simulink model "implementation_deploy_mpc"  (R2024a)
settings: configuration reference "Configuration" (kept outside this file)
undefined symbols (not defined in the file): aceleracao_lateral_max, constans_PID, desired_x, desired_y, max_velocity_longitudinal, pos_theta, pos_x, pos_y, PredictionHorizon, Ts, vel_x
libraries: canmsglib x3, nvidiaCommlib x3, ros2lib x2, svdutilitieslib x1, mpcadaslib x1, drivingvehiclecontroller x1, slpidlib x1
settings Model: DataDictionary=implementacao_deploy.sldd  Creator=helenamandl  LastModifiedBy=thailon
settings ConfigSetRef: SourceName=Configuration

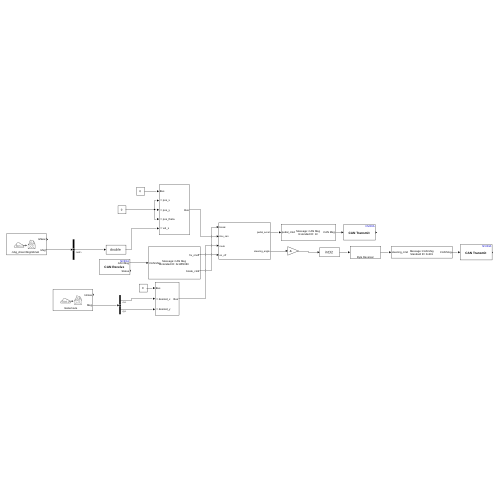
[thumbnail: Simulink's stored preview of the top-level diagram]
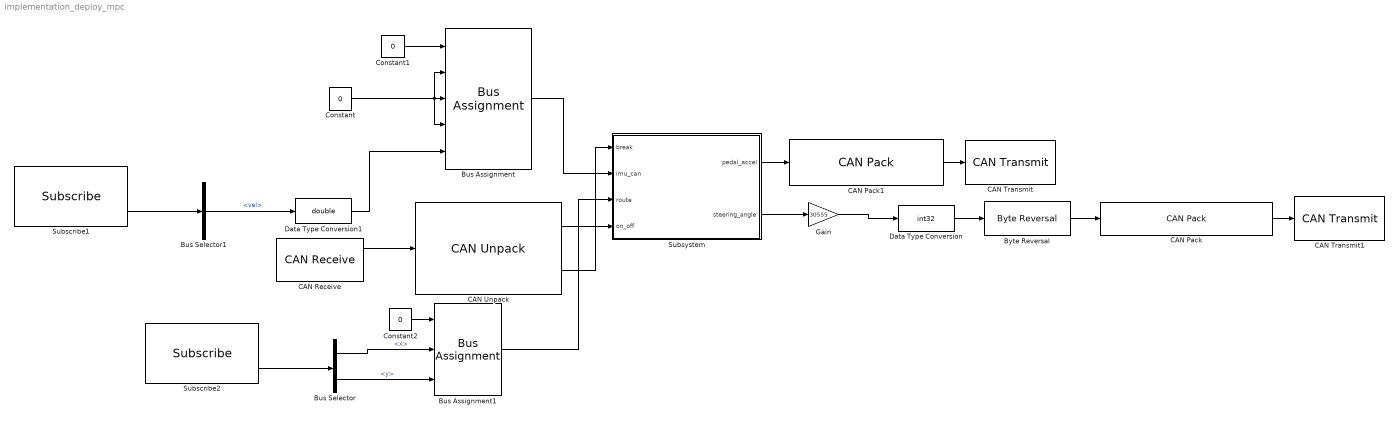
== system implementation_deploy_mpc ==
  Bus Assignment : BusAssignment  AssignedSignals=pos_x,pos_y,pos_theta,vel_x
  Bus Assignment1 : BusAssignment  AssignedSignals=desired_x,desired_y
  Bus Selector : BusSelector  OutputSignals=pose.position.x,pose.position.y
  Bus Selector1 : BusSelector  OutputSignals=vel
  Byte Reversal : svdutilitieslib/Byte Reversal  numInp=1  blockPlatform=arduinoert
      settings: LibrarySourceBlock=mcblib/Signal Management/Byte Reversal
  CAN Pack : canmsglib/CAN Pack  MsgList=(none)  MsgName=CAN Msg  MsgIDType=Standard (11-bit identifier)  MsgIdentifier=0x401  MsgLength=4  Remote=off  ApplyMinMax=off  BusOutput=on  SignalInfo={ 'steering_cmd', '0', '32', 'LE', 'signed', 'Standard', '0', '1', '0', '-Inf', 'Inf' }
      settings: LibrarySourceBlock=c2000lib/Target Communication/CAN Pack  DataFormat=manually specified signals
  CAN Pack1 : canmsglib/CAN Pack  MsgList=(none)  MsgName=CAN Msg  MsgIDType=Extended (29-bit identifier)  MsgIdentifier=13  MsgLength=1  Remote=off  ApplyMinMax=off  BusOutput=on  SignalInfo={ 'pedal_cmd', '0', '8', 'LE', 'unsigned', 'Standard', '0', '1', '0', '0', '100' }
      settings: LibrarySourceBlock=c2000lib/Target Communication/CAN Pack  DataFormat=manually specified signals
  CAN Receive : nvidiaCommlib/CAN Receive  DeviceID=can0  SetupCAN=off  TypeofCAN=Real  OutputDataType=CAN Msg  IdentifierType=Extended (29-bit identifier)  MessageId=0x18ff1080  MsgLength=8  SampleTime=0.005  OutputError=off  OutputRemote=off  SimulateUsing=Code generation
  CAN Transmit : nvidiaCommlib/CAN Transmit  DeviceID=vcan0  SetupCAN=off  TypeofCAN=Real  InputDataType=CAN Msg  BlockingMode_=off  BlockTimeout_=1  OutputStatus=on  IdentifierType=Standard (11-bit identifier)  MessageId=13  MsgLength=8  RemoteFrame=off  SimulateUsing=Code generation
  CAN Transmit1 : nvidiaCommlib/CAN Transmit  DeviceID=vcan0  SetupCAN=off  TypeofCAN=Real  InputDataType=CAN Msg  BlockingMode_=off  BlockTimeout_=1  OutputStatus=on  IdentifierType=Extended (29-bit identifier)  MessageId=0x401  MsgLength=4  RemoteFrame=off  SimulateUsing=Code generation
  CAN Unpack : canmsglib/CAN Unpack  MsgList=(none)  MsgName=CAN Msg  MsgIDType=Extended (29-bit identifier)  MsgIdentifier=0x18ff1080  MsgLength=4  SignalInfo={ 'hv_onoff', '0', '2', 'LE', 'signed', 'Standard', '0', '1', '0', '0', '3'; 'break_cmd', '3', '8', 'LE', 'signed', 'Standard', '1', '1', '0', '0', '255' }  IDPort=off  TimestampPort=off  ErrorPort=off  RemotePort=off  LengthPort=off  StatusPort=off  ApplyMinMax=off
      settings: LibrarySourceBlock=embeddedtargetslib/Host Communication/CAN Unpack
  Constant : Constant  Value=0
  Constant1 : Constant  Value=0  OutDataTypeStr=Bus: bus_imu
  Constant2 : Constant  Value=0  OutDataTypeStr=Bus: bus_route
  Data Type Conversion : DataTypeConversion  OutDataTypeStr=int32  SaturateOnIntegerOverflow=off  RndMeth=Floor
  Data Type Conversion1 : DataTypeConversion  OutDataTypeStr=double  SaturateOnIntegerOverflow=off  RndMeth=Floor
  Gain : Gain  Gain=30555
  Subscribe1 : ros2lib/Subscribe  topicSource=Specify your own  topic=/sbg_driver/SbgOdoVel  messageType=sbg_driver/SbgOdoVel  sampleTime=ts_ros2  QOSHistory=Keep last  QOSDepth=10  QOSReliability=Reliable  QOSDurability=Volatile  QOSDeadline=Inf  QOSLifespan=Inf  QOSLiveliness=Automatic  QOSLeaseDuration=Inf  QOSAvoidROSNamespaceConventions=off
  Subscribe2 : ros2lib/Subscribe  topicSource=Specify your own  topic=/teste/route  messageType=geometry_msgs/PoseStamped  sampleTime=ts_ros2  QOSHistory=Keep last  QOSDepth=10  QOSReliability=Reliable  QOSDurability=Volatile  QOSDeadline=Inf  QOSLifespan=Inf  QOSLiveliness=Automatic  QOSLeaseDuration=Inf  QOSAvoidROSNamespaceConventions=off
  Subsystem : Subsystem
  wires:
  CAN Pack/1 -> CAN Transmit1/1
  Data Type Conversion/1 -> Byte Reversal/1
  Subsystem/1(pedal_accel) -> CAN Pack1/1
  Bus Assignment1/1 -> Subsystem/3(route)
  CAN Unpack/1 -> Subsystem/4(on_off)
  Bus Assignment/1 -> Subsystem/2(imu_can)
  Byte Reversal/1 -> CAN Pack/1
  Bus Selector/2 -> Bus Assignment1/3  "<y>"
  Subscribe1/2 -> Bus Selector1/1
  Bus Selector1/1 -> Data Type Conversion1/1  "<vel>"
  CAN Pack1/1 -> CAN Transmit/1
  Constant2/1 -> Bus Assignment1/1
  CAN Unpack/2 -> Subsystem/1(break)
  Subscribe2/2 -> Bus Selector/1
  Gain/1 -> Data Type Conversion/1
  Subsystem/2(steering_angle) -> Gain/1
  Data Type Conversion1/1 -> Bus Assignment/5
  Bus Selector/1 -> Bus Assignment1/2  "<x>"
  Constant1/1 -> Bus Assignment/1
  CAN Receive/1 -> CAN Unpack/1
  Constant/1 -> Bus Assignment/2, Bus Assignment/4, Bus Assignment/3

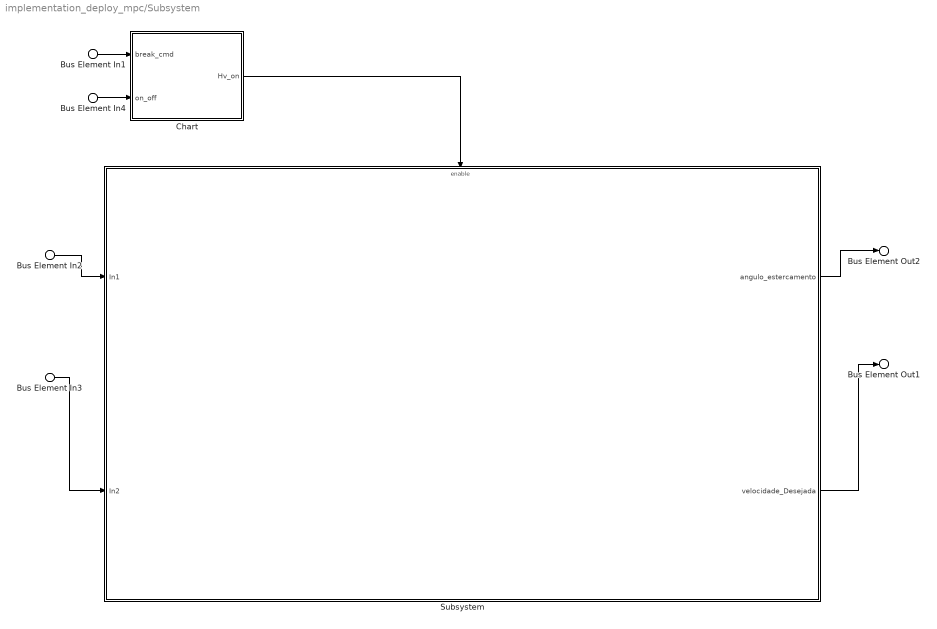
== system implementation_deploy_mpc/Subsystem ==
  Bus Element In1 : Inport  PortName=break
  Bus Element In2 : Inport  Port=2  PortName=imu_can
  Bus Element In3 : Inport  Port=3  PortName=route
  Bus Element In4 : Inport  Port=4  PortName=on_off
  Chart : Stateflow chart  TreatAsAtomicUnit=on
  Subsystem : Subsystem
  Bus Element Out1 : Outport  PortName=pedal_accel
  Bus Element Out2 : Outport  Port=2  PortName=steering_angle
  wires:
  Bus Element In1/1 -> Chart/1(break_cmd)
  Subsystem/1(angulo_estercamento) -> Bus Element Out2/1
  Subsystem/2(velocidade_Desejada) -> Bus Element Out1/1
  Chart/1(Hv_on) -> Subsystem/Enable
  Bus Element In4/1 -> Chart/2(on_off)
  Bus Element In2/1 -> Subsystem/1(In1)
  Bus Element In3/1 -> Subsystem/2(In2)

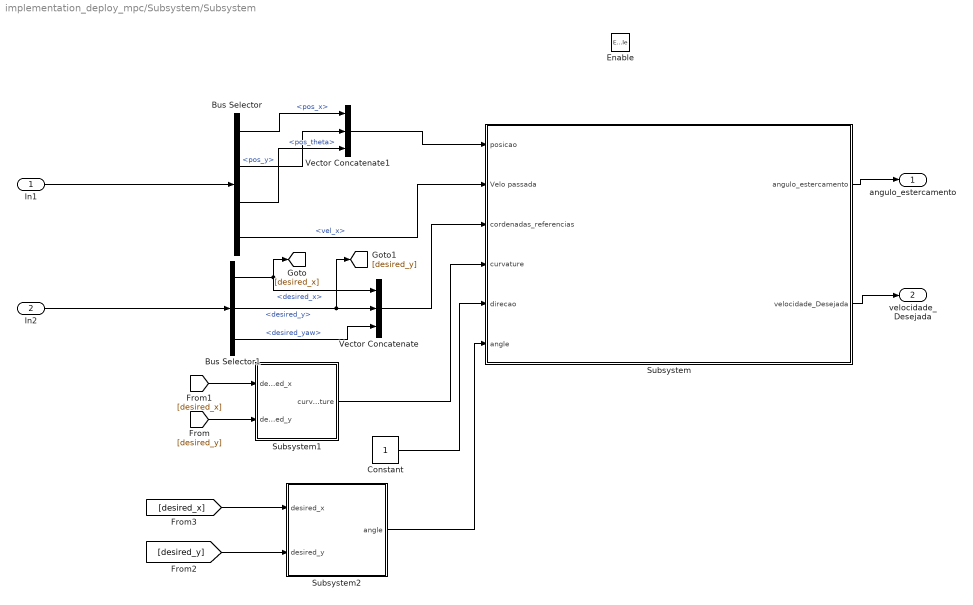
== system implementation_deploy_mpc/Subsystem/Subsystem ==
  In1 : Inport
  In2 : Inport  Port=2
  Enable : EnablePort
  Bus Selector : BusSelector  OutputSignals=pos_x,pos_y,pos_theta,vel_x
  Bus Selector1 : BusSelector  OutputSignals=desired_x,desired_y,desired_yaw
  Constant : Constant
  Subsystem : Subsystem
  Subsystem1 : Subsystem
  Subsystem2 : Subsystem
  Vector Concatenate : Concatenate  NumInputs=3
  Vector Concatenate1 : Concatenate  NumInputs=3
  angulo_estercamento : Outport
  velocidade_Desejada : Outport  Port=2
  wires:
  [desired_y] -> Subsystem1/2(desired_y)
  Bus Selector/4 -> Subsystem/2(Velo passada)  "<vel_x>"
  Subsystem/1(angulo_estercamento) -> angulo_estercamento/1
  Bus Selector/1 -> Vector Concatenate1/1  "<pos_x>"
  Bus Selector1/1 -> Vector Concatenate/1, [desired_x]  "<desired_x>"
  Bus Selector/2 -> Vector Concatenate1/2  "<pos_y>"
  [desired_x] -> Subsystem1/1(desired_x)
  In1/1 -> Bus Selector/1
  Bus Selector1/2 -> Vector Concatenate/2, [desired_y]  "<desired_y>"
  Vector Concatenate/1 -> Subsystem/3(cordenadas_referencias)
  Bus Selector1/3 -> Vector Concatenate/3  "<desired_yaw>"
  In2/1 -> Bus Selector1/1
  Bus Selector/3 -> Vector Concatenate1/3  "<pos_theta>"
  Subsystem/2(velocidade_Desejada) -> velocidade_Desejada/1
  Vector Concatenate1/1 -> Subsystem/1(posicao)
  Constant/1 -> Subsystem/5(direcao)
  Subsystem1/1(curvature) -> Subsystem/4(curvature)
  [desired_x] -> Subsystem2/1(desired_x)
  [desired_y] -> Subsystem2/2(desired_y)
  Subsystem2/1(angle) -> Subsystem/6(angle)

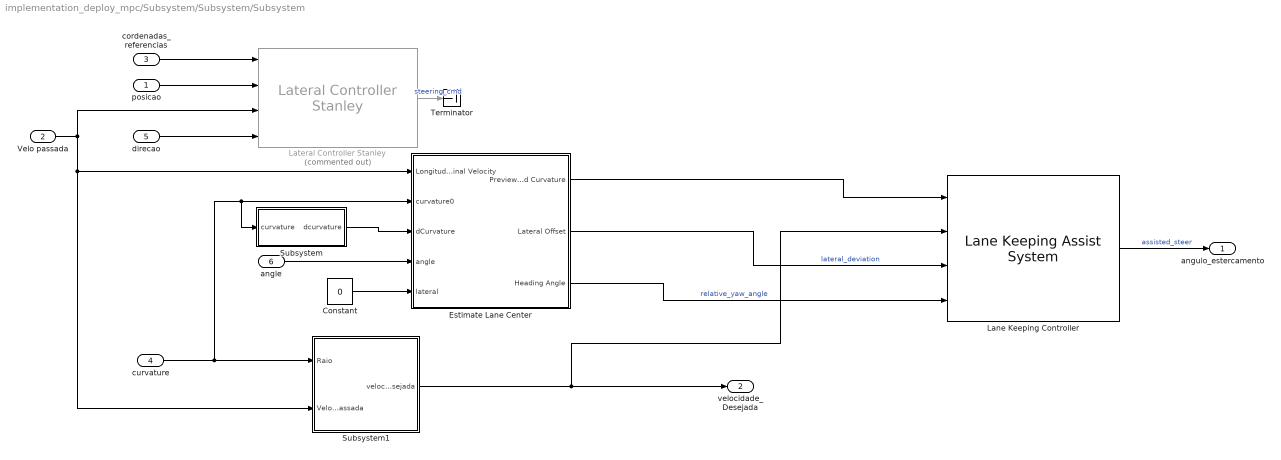
== system implementation_deploy_mpc/Subsystem/Subsystem/Subsystem ==
  posicao : Inport
  Velo passada : Inport  Port=2
  cordenadas_referencias : Inport  Port=3
  curvature : Inport  Port=4
  direcao : Inport  Port=5
  angle : Inport  Port=6
  Constant : Constant  Value=0
  Estimate Lane Center : Subsystem  VariantControl=v2
  Lane Keeping Controller : mpcadaslib/Lane Keeping Assist System  ModelType=Use vehicle parameters  VehicleMass=m  VehicleYawInertia=Iz  LengthToFront=lf  LengthToRear=lr  FrontTireStiffness=Cf  RearTireStiffness=Cr  EgoModelMatrixA=[-4.4021 ,-12.4603;1.3913,-5.1868]  EgoModelMatrixB=[24.1270;15.8609]  EgoModelMatrixC=[1,0;0,1]  InitialLongVel=v0_ego  TransportLag=0  MinSteering=-0.5  umin_ext=off  MaxSteering=0.5  umax_ext=off  Ts=Ts  PredictionHorizon=PredictionHorizon  ControllerBehavior=0.200  suboptimal=off  maxiter=10  datatypeopt=single  optmode=off  trackmode=off
  Lateral Controller Stanley : drivingvehiclecontroller/Lateral Controller Stanley  Commented=on  ModelType=Kinematic bicycle model  PositionGainF=stanley_kpfw  PositionGainR=stanley_kprv  YawRateGain=1  DelayGain=0.2  VehicleMass=230  Lf=1.4  Lr=1.6  TireStiffness=12e3  Wheelbase=wheelbase  MaxSteeringAngle=max_steering_angle
  Subsystem : Subsystem
  Subsystem1 : Subsystem
  Terminator : Terminator
  angulo_estercamento : Outport  OutMax=[0]  PortDimensions=1
  velocidade_Desejada : Outport  Port=2
  wires:
  direcao/1 -> Lateral Controller Stanley/4
  posicao/1 -> Lateral Controller Stanley/2
  cordenadas_referencias/1 -> Lateral Controller Stanley/1
  Subsystem1/1(velocidade_desejada) -> Lane Keeping Controller/2, velocidade_Desejada/1
  Velo passada/1 -> Subsystem1/2(Velo passada), Estimate Lane Center/1(Longitudinal Velocity), Lateral Controller Stanley/3
  curvature/1 -> Subsystem1/1(Raio), Subsystem/1(curvature), Estimate Lane Center/2(curvature0)
  Estimate Lane Center/3(Heading Angle) -> Lane Keeping Controller/4  "relative_yaw_angle"
  Estimate Lane Center/1(Previewed Curvature) -> Lane Keeping Controller/1
  Lane Keeping Controller/1 -> angulo_estercamento/1  "assisted_steer"
  Estimate Lane Center/2(Lateral Offset) -> Lane Keeping Controller/3  "lateral_deviation"
  angle/1 -> Estimate Lane Center/4(angle)
  Constant/1 -> Estimate Lane Center/5(lateral)
  Subsystem/1(dcurvature) -> Estimate Lane Center/3(dCurvature)
  Lateral Controller Stanley/1 -> Terminator/1  "steering_cmd"

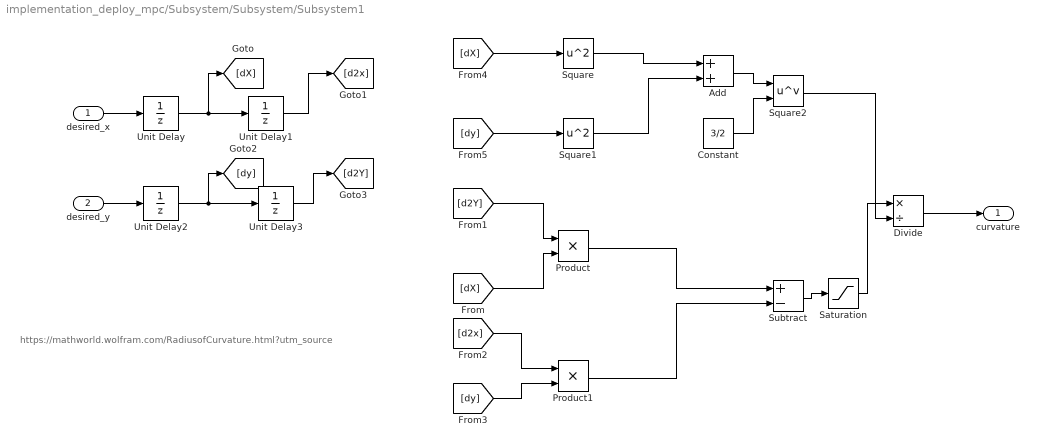
== system implementation_deploy_mpc/Subsystem/Subsystem/Subsystem1 ==
  note: https://mathworld.wolfram.com/RadiusofCurvature.html?utm_source
  desired_x : Inport
  desired_y : Inport  Port=2
  Add : Sum
  Constant : Constant  Value=3/2
  Divide : Product  Inputs=*/
  Product : Product
  Product1 : Product
  Saturation : Saturate  UpperLimit=10000  LowerLimit=0.00001
  Square : Math  Operator=square
  Square1 : Math  Operator=square
  Square2 : Math  Operator=pow
  Subtract : Sum  Inputs=+-
  Unit Delay{,1..3} (4 alike) : UnitDelay  SampleTime=-1  HasFrameUpgradeWarning=on
  curvature : Outport
  wires:
  [dX] -> Square/1
  [d2x] -> Product1/1
  desired_x/1 -> Unit Delay/1
  [dy] -> Product1/2
  Product/1 -> Subtract/1
  Unit Delay1/1 -> [d2x]
  Add/1 -> Square2/1
  Unit Delay/1 -> [dX], Unit Delay1/1
  Square1/1 -> Add/2
  [d2Y] -> Product/1
  [dy] -> Square1/1
  Product1/1 -> Subtract/2
  [dX] -> Product/2
  desired_y/1 -> Unit Delay2/1
  Unit Delay2/1 -> [dy], Unit Delay3/1
  Constant/1 -> Square2/2
  Unit Delay3/1 -> [d2Y]
  Divide/1 -> curvature/1
  Square2/1 -> Divide/2
  Subtract/1 -> Saturation/1
  Saturation/1 -> Divide/1
  Square/1 -> Add/1

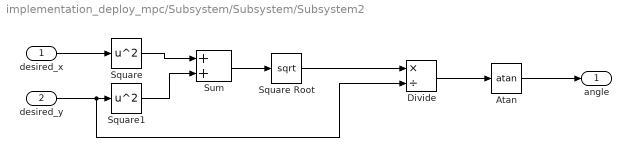
== system implementation_deploy_mpc/Subsystem/Subsystem/Subsystem2 ==
  desired_x : Inport
  desired_y : Inport  Port=2
  Atan : Trigonometry  Operator=atan
  Divide : Product  Inputs=*/
  Square : Math  Operator=square
  Square Root : Sqrt
  Square1 : Math  Operator=square
  Sum : Sum
  angle : Outport
  wires:
  desired_x/1 -> Square/1
  desired_y/1 -> Divide/2, Square1/1
  Square/1 -> Sum/1
  Square1/1 -> Sum/2
  Sum/1 -> Square Root/1
  Square Root/1 -> Divide/1
  Divide/1 -> Atan/1
  Atan/1 -> angle/1

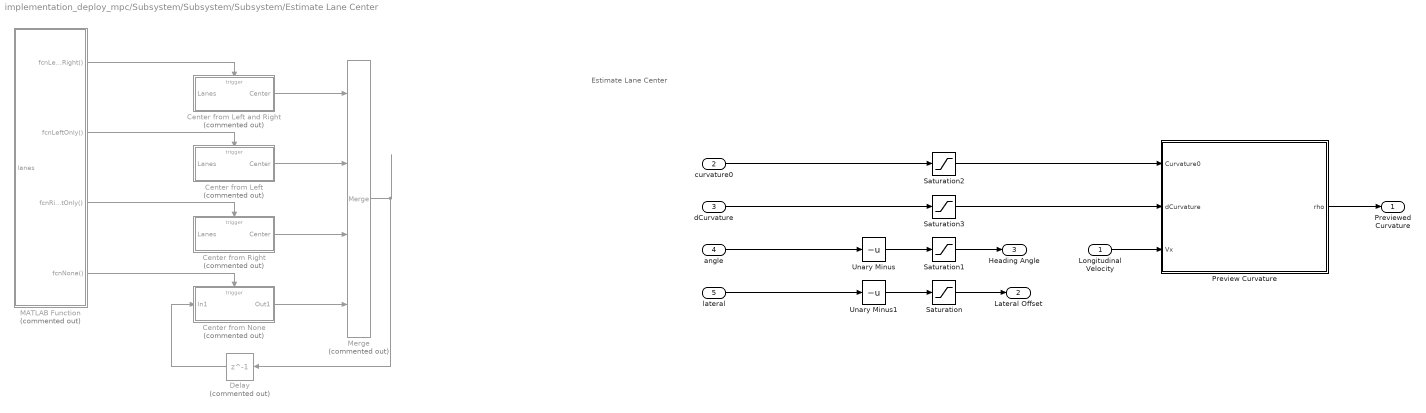
== system implementation_deploy_mpc/Subsystem/Subsystem/Subsystem/Estimate Lane Center ==
  note: Estimate Lane Center
  Longitudinal Velocity : Inport  OutDataTypeStr=single
  curvature0 : Inport  Port=2
  dCurvature : Inport  Port=3
  angle : Inport  Port=4
  lateral : Inport  Port=5
  Center from Left : Subsystem  Commented=on  TreatAsAtomicUnit=on
  Center from Left and Right : Subsystem  Commented=on  TreatAsAtomicUnit=on
  Center from None : Subsystem  Commented=on  TreatAsAtomicUnit=on
  Center from Right : Subsystem  Commented=on  TreatAsAtomicUnit=on
  Delay : Delay  Commented=on  DelayLength=1
  MATLAB Function : MATLAB Function  Commented=on  TreatAsAtomicUnit=on
  Merge : Merge  Commented=on  Inputs=4
  Preview Curvature : MATLAB Function  TreatAsAtomicUnit=on  SystemSampleTime=Ts
  Saturation : Saturate
  Saturation1 : Saturate  UpperLimit=0.6  LowerLimit=-0.6
  Saturation2 : Saturate  UpperLimit=0.15  LowerLimit=-0.15
  Saturation3 : Saturate  UpperLimit=0.06  LowerLimit=-0.06
  Unary Minus : UnaryMinus
  Unary Minus1 : UnaryMinus
  Previewed Curvature : Outport  VectorParamsAs1DForOutWhenUnconnected=off
  Lateral Offset : Outport  Port=2  VectorParamsAs1DForOutWhenUnconnected=off
  Heading Angle : Outport  Port=3  VectorParamsAs1DForOutWhenUnconnected=off
  wires:
  angle/1 -> Unary Minus/1
  lateral/1 -> Unary Minus1/1
  Unary Minus1/1 -> Saturation/1
  curvature0/1 -> Saturation2/1
  dCurvature/1 -> Saturation3/1
  Longitudinal Velocity/1 -> Preview Curvature/3(Vx)
  Preview Curvature/1(rho) -> Previewed Curvature/1
  Unary Minus/1 -> Saturation1/1
  Saturation/1 -> Lateral Offset/1
  Saturation1/1 -> Heading Angle/1
  Saturation2/1 -> Preview Curvature/1(Curvature0)
  Saturation3/1 -> Preview Curvature/2(dCurvature)
  Merge/1 -> Delay/1
  Center from Left/1(Center) -> Merge/2
  MATLAB Function/4(fcnNone()) -> Center from None/Trigger
  MATLAB Function/3(fcnRightOnly()) -> Center from Right/Trigger
  Center from Left and Right/1(Center) -> Merge/1
  Delay/1 -> Center from None/1(In1)
  MATLAB Function/1(fcnLeftAndRight()) -> Center from Left and Right/Trigger
  Center from None/1(Out1) -> Merge/4
  MATLAB Function/2(fcnLeftOnly()) -> Center from Left/Trigger
  Center from Right/1(Center) -> Merge/3

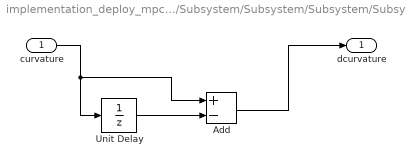
== system implementation_deploy_mpc/Subsystem/Subsystem/Subsystem/Subsystem ==
  curvature : Inport
  Add : Sum  Inputs=+-
  Unit Delay : UnitDelay  SampleTime=-1  HasFrameUpgradeWarning=on
  dcurvature : Outport
  wires:
  curvature/1 -> Add/1, Unit Delay/1
  Unit Delay/1 -> Add/2
  Add/1 -> dcurvature/1

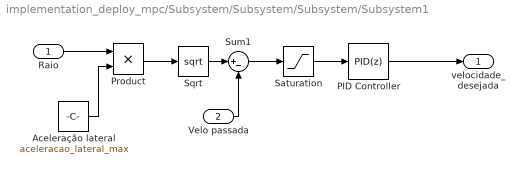
== system implementation_deploy_mpc/Subsystem/Subsystem/Subsystem/Subsystem1 ==
  Raio : Inport
  Velo passada : Inport  Port=2
  Aceleração lateral : Constant  Value=aceleracao_lateral_max
  PID Controller : slpidlib/PID Controller  Controller=PID  Form=Parallel  TimeDomain=Discrete-time  UseExternalTs=off  SampleTime=-1  IntegratorMethod=Forward Euler  FilterMethod=Forward Euler  ControllerParametersSource=internal  P=constans_PID(1)  I=constans_PID(2)  UseKiTs=off  D=constans_PID(3)  UseExternalDerivativeSource=off  N=constans_PID(4)  UseFilter=on  TunerSelectOption=Transfer Function Based (PID Tuner App)  InitialConditionSource=internal  InitialConditionForIntegrator=0  InitialConditionForFilter=0  DifferentiatorICPrevScaledInput=0  ExternalReset=none  TrackingMode=off  Kt=1  LimitOutput=off  SatLimitsSource=internal  UpperSaturationLimit=12  LowerSaturationLimit=-12  LinearizeAsGain=on  AntiWindupMode=none  Kb=1  LimitIntegrator=off  UpperIntegratorSaturationLimit=inf  LowerIntegratorSaturationLimit=-inf  POutMin=[]  POutMax=[]  IOutMin=[]  IOutMax=[]  DOutMin=[]  DOutMax=[]  NOutMin=[]  NOutMax=[]  SumOutMin=[]  SumOutMax=[]  SaturationOutMin=[]  SaturationOutMax=[]  PParamMin=[]  PParamMax=[]  IParamMin=[]  IParamMax=[]  DParamMin=[]  DParamMax=[]  NParamMin=[]  NParamMax=[]  KbParamMin=[]  KbParamMax=[]  KtParamMin=[]  KtParamMax=[]  KbOutMin=[]  KbOutMax=[]  KtOutMin=[]  KtOutMax=[]  IntegratorOutMin=[]  IntegratorOutMax=[]  FilterOutMin=[]  FilterOutMax=[]  SumI1OutMin=[]  SumI1OutMax=[]  SumI2OutMin=[]  SumI2OutMax=[]  SumI3OutMin=[]  SumI3OutMax=[]  SumI4OutMin=[]  SumI4OutMax=[]  SumDOutMin=[]  SumDOutMax=[]  DifferentiatorOutMin=[]  DifferentiatorOutMax=[]  FilterDiffOutCoefMin=[]  FilterDiffOutCoefMax=[]  ReciprocalOutMin=[]  ReciprocalOutMax=[]  SumDenOutMin=[]  SumDenOutMax=[]  SumNumOutMin=[]  SumNumOutMax=[]  DivideOutMin=[]  DivideOutMax=[]  UdiffTsProdOutMin=[]  UdiffTsProdOutMax=[]  NTsProdOutMin=[]  NTsProdOutMax=[]  UintegralTsProdOutMin=[]  UintegralTsProdOutMax=[]  UngainTsProdOutMin=[]  UngainTsProdOutMax=[]  ClampingZeroOutDataTypeStr=Inherit: Inherit via back propagation  ClampingZeroOutMin=[]  ClampingZeroOutMax=[]  FilterDenConstantOutDataTypeStr=Inherit: Inherit via back propagation  FilterDenConstantOutMin=[]  FilterDenConstantOutMax=[]  PCopyOutDataTypeStr=Inherit: Inherit via back propagation  PCopyOutMin=[]  PCopyOutMax=[]  NCopyOutDataTypeStr=Inherit: Inherit via back propagation  NCopyOutMin=[]  NCopyOutMax=[]  IntegratorContinuousStateAttributes=''  IntegratorStateMustResolveToSignalObject=off  IntegratorRTWStateStorageClass=Auto  FilterContinuousStateAttributes=''  FilterStateMustResolveToSignalObject=off  FilterRTWStateStorageClass=Auto  ParallelPVariant=InternalParameters  IdealPVariant=Disabled  IVariant=InternalParameters  DVariant=InternalParameters  IntegratorVariant=Discrete  SatVariant=Disabled  AWVariant=Passthrough  PCopyVariant=Disabled  TRVariant=Disabled  FdbkBlocksVariant=Forward  IdealPFdbkVariant=Disabled  SatFdbkVariant=Disabled  DerivativeFilterVariant=ForwardEulerFilter  NVariant=InternalParameters  NCopyVariant=Disabled  FilterICVariant=InternalICsFilter  IntegratorICVariant=InternalICs  ExternalResetVariant=Disabled  TRSumVariant=Passthrough  SumFdbkVariant=Disabled  SumVariant=Sum_PID  TsampFilterVariant=InternalTs  TsampNgainVariant=Passthrough  TsampIntegralVariant=Disabled_SignalSpec  ExternalSaturationOutDataTypeStr=Inherit: Same as second input  DerivativeSourceVariant=ErrorSignal
  Product : Product
  Saturation : Saturate  UpperLimit=max_velocity_longitudinal  LowerLimit=0
      settings: AttributesFormatString=Velocidade maxima do carro=%<UpperLimit>
  Sqrt : Sqrt
  Sum1 : Sum  Inputs=|+-
  velocidade_desejada : Outport
  wires:
  Saturation/1 -> PID Controller/1
  Sum1/1 -> Saturation/1
  PID Controller/1 -> velocidade_desejada/1
  Product/1 -> Sqrt/1
  Aceleração lateral/1 -> Product/2
  Sqrt/1 -> Sum1/1
  Raio/1 -> Product/1
  Velo passada/1 -> Sum1/2

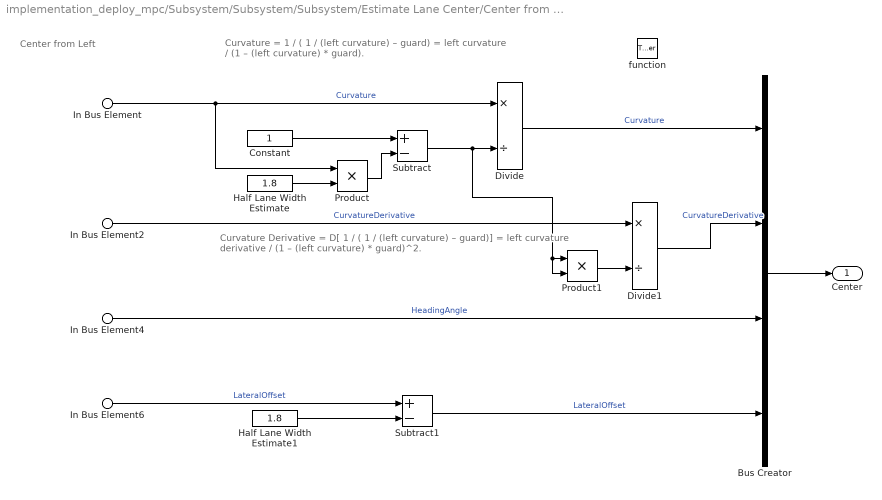
== system implementation_deploy_mpc/Subsystem/Subsystem/Subsystem/Estimate Lane Center/Center from Left ==
  note: Curvature
      | = 1 / ( 1 / (left curvature) – guard)
      | = left curvature / (1 – (left curvature) * guard).
  note: Center from Left
  note: Curvature Derivative
      | = D[ 1 / ( 1 / (left curvature) – guard)]
      | = left curvature derivative / (1 – (left curvature) * guard)^2.
  In Bus Element : Inport  PortName=Lanes  Element=Left.Curvature
  In Bus Element2 : Inport  PortName=Lanes  Element=Left.CurvatureDerivative
  In Bus Element4 : Inport  PortName=Lanes  Element=Left.HeadingAngle
  In Bus Element6 : Inport  PortName=Lanes  Element=Left.LateralOffset
  function : TriggerPort  TriggerType=function-call  VariantControl=Variant
  Bus Creator : BusCreator  Inputs=4
  Constant : Constant  OutDataTypeStr=Inherit: Inherit via back propagation
  Divide : Product  Inputs=*/
  Divide1 : Product  Inputs=*/
  Half Lane Width Estimate : Constant  Value=1.8  OutDataTypeStr=Inherit: Inherit via back propagation
  Half Lane Width Estimate1 : Constant  Value=1.8  OutDataTypeStr=Inherit: Inherit via back propagation
  Product : Product
  Product1 : Product
  Subtract : Sum  Inputs=+-
  Subtract1 : Sum  Inputs=+-
  Center : Outport  VectorParamsAs1DForOutWhenUnconnected=off
  wires:
  Bus Creator/1 -> Center/1
  Divide1/1 -> Bus Creator/2  "CurvatureDerivative"
  Divide/1 -> Bus Creator/1  "Curvature"
  In Bus Element4/1 -> Bus Creator/3  "HeadingAngle"
  Subtract1/1 -> Bus Creator/4  "LateralOffset"
  In Bus Element/1 -> Product/1, Divide/1  "Curvature"
  Subtract/1 -> Product1/2, Product1/1, Divide/2
  Half Lane Width Estimate/1 -> Product/2
  Constant/1 -> Subtract/1
  In Bus Element2/1 -> Divide1/1  "CurvatureDerivative"
  Product1/1 -> Divide1/2
  In Bus Element6/1 -> Subtract1/1  "LateralOffset"
  Half Lane Width Estimate1/1 -> Subtract1/2
  Product/1 -> Subtract/2

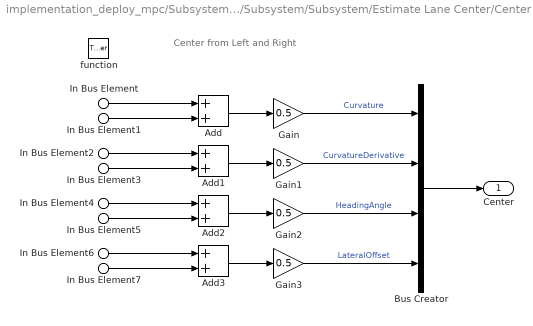
== system implementation_deploy_mpc/Subsystem/Subsystem/Subsystem/Estimate Lane Center/Center from Left and Right ==
  note: Center from Left and Right
  In Bus Element : Inport  PortName=Lanes  Element=Left.Curvature
  In Bus Element2 : Inport  PortName=Lanes  Element=Left.CurvatureDerivative
  In Bus Element4 : Inport  PortName=Lanes  Element=Left.HeadingAngle
  In Bus Element6 : Inport  PortName=Lanes  Element=Left.LateralOffset
  In Bus Element1 : Inport  PortName=Lanes  Element=Right.Curvature
  In Bus Element3 : Inport  PortName=Lanes  Element=Right.CurvatureDerivative
  In Bus Element5 : Inport  PortName=Lanes  Element=Right.HeadingAngle
  In Bus Element7 : Inport  PortName=Lanes  Element=Right.LateralOffset
  function : TriggerPort  TriggerType=function-call  VariantControl=Variant
  Add{,1..3} (4 alike) : Sum
  Bus Creator : BusCreator  Inputs=4
  Gain{,1..3} (4 alike) : Gain  Gain=0.5
  Center : Outport  VectorParamsAs1DForOutWhenUnconnected=off
  wires:
  Add/1 -> Gain/1
  Gain/1 -> Bus Creator/1  "Curvature"
  Add1/1 -> Gain1/1
  Gain1/1 -> Bus Creator/2  "CurvatureDerivative"
  Add2/1 -> Gain2/1
  Gain2/1 -> Bus Creator/3  "HeadingAngle"
  Add3/1 -> Gain3/1
  Gain3/1 -> Bus Creator/4  "LateralOffset"
  Bus Creator/1 -> Center/1
  In Bus Element/1 -> Add/1
  In Bus Element1/1 -> Add/2
  In Bus Element2/1 -> Add1/1
  In Bus Element3/1 -> Add1/2
  In Bus Element4/1 -> Add2/1
  In Bus Element5/1 -> Add2/2
  In Bus Element7/1 -> Add3/2
  In Bus Element6/1 -> Add3/1

== system implementation_deploy_mpc/Subsystem/Subsystem/Subsystem/Estimate Lane Center/Center from None ==
  In1 : Inport
  function : TriggerPort  TriggerType=function-call  VariantControl=Variant
  Out1 : Outport  VectorParamsAs1DForOutWhenUnconnected=off
  wires:
  In1/1 -> Out1/1

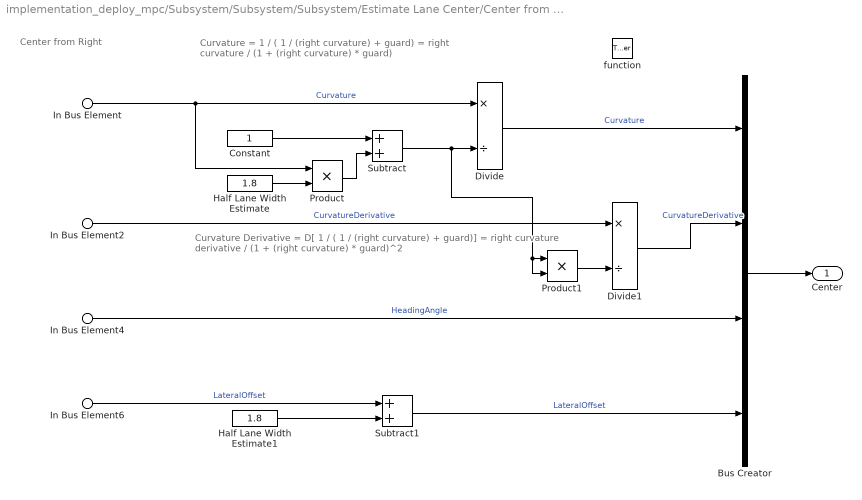
== system implementation_deploy_mpc/Subsystem/Subsystem/Subsystem/Estimate Lane Center/Center from Right ==
  note: Center from Right
  note: Curvature
      | = 1 / ( 1 / (right curvature) + guard)
      | = right curvature / (1 + (right curvature) * guard)
  note: Curvature Derivative
      | = D[ 1 / ( 1 / (right curvature) + guard)]
      | = right curvature derivative / (1 + (right curvature) * guard)^2
  In Bus Element : Inport  PortName=Lanes  Element=Right.Curvature
  In Bus Element2 : Inport  PortName=Lanes  Element=Right.CurvatureDerivative
  In Bus Element4 : Inport  PortName=Lanes  Element=Right.HeadingAngle
  In Bus Element6 : Inport  PortName=Lanes  Element=Right.LateralOffset
  function : TriggerPort  TriggerType=function-call  VariantControl=Variant
  Bus Creator : BusCreator  Inputs=4
  Constant : Constant  OutDataTypeStr=Inherit: Inherit via back propagation
  Divide : Product  Inputs=*/
  Divide1 : Product  Inputs=*/
  Half Lane Width Estimate : Constant  Value=1.8  OutDataTypeStr=Inherit: Inherit via back propagation
  Half Lane Width Estimate1 : Constant  Value=1.8  OutDataTypeStr=Inherit: Inherit via back propagation
  Product : Product
  Product1 : Product
  Subtract : Sum
  Subtract1 : Sum
  Center : Outport  VectorParamsAs1DForOutWhenUnconnected=off
  wires:
  In Bus Element2/1 -> Divide1/1  "CurvatureDerivative"
  Divide1/1 -> Bus Creator/2  "CurvatureDerivative"
  Product1/1 -> Divide1/2
  In Bus Element4/1 -> Bus Creator/3  "HeadingAngle"
  Half Lane Width Estimate1/1 -> Subtract1/2
  In Bus Element6/1 -> Subtract1/1  "LateralOffset"
  Divide/1 -> Bus Creator/1  "Curvature"
  Subtract1/1 -> Bus Creator/4  "LateralOffset"
  Bus Creator/1 -> Center/1
  In Bus Element/1 -> Product/1, Divide/1  "Curvature"
  Subtract/1 -> Product1/2, Product1/1, Divide/2
  Constant/1 -> Subtract/1
  Product/1 -> Subtract/2
  Half Lane Width Estimate/1 -> Product/2

== stateflow chart implementation_deploy_mpc/Subsystem/Chart ==
  state Idle
  state HV
    entry:
    Hv_on = 1;
  (default) -> Idle
  Idle -> HV : [on_off==true]
  HV -> Idle : [(on_off == false) || (break_cmd == true) ]
  data: break_cmd input; on_off input; Hv_on output

== matlab function implementation_deploy_mpc/Subsystem/Subsystem/Subsystem/Estimate Lane Center/MATLAB Function ==
  data: lanes input
  events: fcnLeftAndRight output FUNCTION_CALL_EVENT; fcnLeftOnly output FUNCTION_CALL_EVENT; fcnRightOnly output FUNCTION_CALL_EVENT; fcnNone output FUNCTION_CALL_EVENT
function fcn(lanes)

leftStrength  = lanes.Left.Strength;
rightStrength = lanes.Right.Strength;

if (leftStrength > 0) && (rightStrength > 0)
   fcnLeftAndRight();
   
elseif leftStrength > 0
    fcnLeftOnly();
    
elseif rightStrength > 0
    fcnRightOnly();
    
else
    fcnNone();
end

== matlab function implementation_deploy_mpc/Subsystem/Subsystem/Subsystem/Estimate Lane Center/Preview Curvature ==
  data: rho output; Curvature0 input; dCurvature input; Vx input; Ts parameter; PredictionHorizon parameter
function rho = predictCurvature(Curvature0,dCurvature,Vx, Ts, PredictionHorizon)
% Curvature0 = initial curvature per unit length                  [1/m]
% dCurvature = (constant) derivative of curvature per unit length [1/m^2]
% CurvatureLength = length for which the clothoid model is valid [m]
% Vx = speed of vehicle

% We want to export a set of curvatures at a uniform sample time ahead.
% t is this vector which goes up to 1 second in the future or having
% enough time to reach the known length in curvature (whichever is smaller)

% To enable truncation by curvelength, mark output "rho" as varsize
%t = 0:Ts:min(1,CurvatureLength/Vx);

t = zeros(PredictionHorizon+1,1);
for i=1:numel(t)
    t(i) = (i-1).*Ts;
end

% We compute the curvature vector rho(t) using the specified clothoid model
rho = Curvature0 + dCurvature*Vx*t;
